simulink model "TDPA"  (R2013a)
settings: Solver=ode3  StartTime=0.0  StopTime=inf  FixedStep=1e-3  RelTol=1e-3
undefined symbols (not defined in the file or in its folder): bDevice, bWall, DBPf, DBPv, kc, Kd, Kp, kWall, mc, mDevice, nWall, POPCM_off, POPCS_off, pos, T1, T2, tSampling, xWall
libraries: quarc_library x2
settings Model: SimulationMode=external  Creator=thaole910  LastModifiedBy=Mech430
settings SolverCC: PositivePriorityOrder=on
settings DebuggingCC: FrameProcessingCompatibilityMsg=error
settings RTWCC: SystemTargetFile=quarc_win64.tlc  TemplateMakefile=quarc_default_tmf  Description=QUARC Win64 Target
settings STFCustomTargetCC: TargetPreCompLibLocation=C:\PROGRA~3\QUARC\lib\2015b\win64\release  CodeReplacementLibrary=C89/C90 (ANSI)  ConcurrentExecutionCompliant=on  GRTInterface=on  SystemTargetFile=quarc_win64.tlc
settings GRTTargetCC: TargetPreCompLibLocation=C:\PROGRA~3\QUARC\lib\2015b\win64\release  CodeReplacementLibrary=C89/C90 (ANSI)  ParMdlRefBuildCompliant=off  CompOptLevelCompliant=off  GeneratePreprocessorConditionals=Use local settings  CombineOutputUpdateFcns=off  MatFileLogging=off  GRTInterface=on  ExtMode=on  ExtModeMexFile=quarc_comm

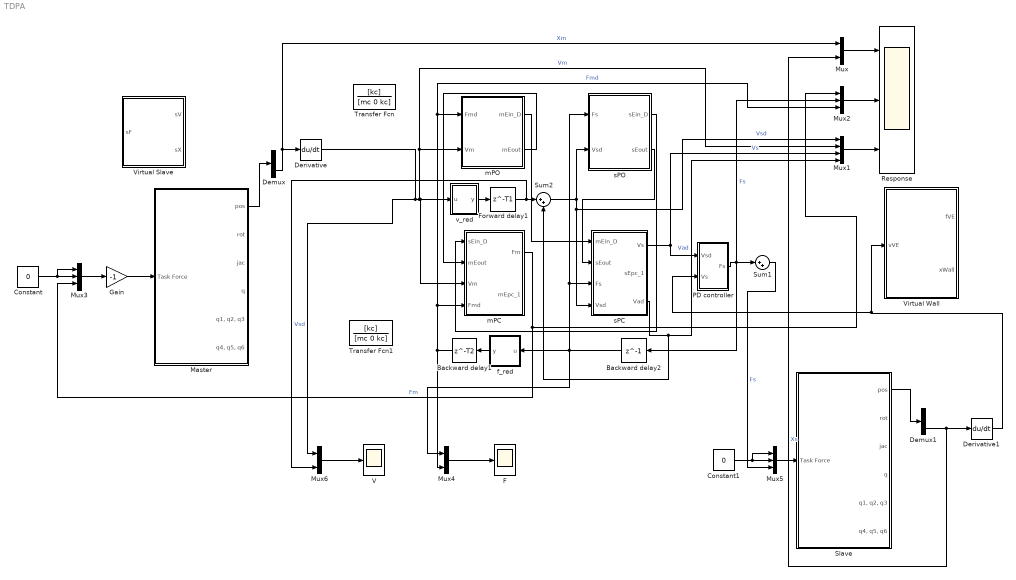
== system TDPA ==
  Backward delay1 : Delay  DelayLength=T2  InitialCondition=0  SampleTime=tSampling
  Backward delay2 : Delay  DelayLength=1  InitialCondition=0  SampleTime=tSampling
  Constant : Constant  Value=0
  Constant1 : Constant  Value=0
  Demux : Demux  Outputs=3
  Demux1 : Demux  Outputs=3
  Derivative : Derivative
  Derivative1 : Derivative
  F : Scope
      settings: TimeRange=100  ShowLegends=on  MaxDataPoints=5000  SaveToWorkspace=off  SaveName=F1  YMin=-4.35585  YMax=15.33258  SampleTime=-1  DataFormat=Array
  Forward delay1 : Delay  DelayLength=T1  InitialCondition=0  SampleTime=tSampling
  Gain : Gain  Gain=-1
  Master : Subsystem
  Mux : Mux  Inputs=2
  Mux1 : Mux
  Mux2 : Mux  Inputs=3
  Mux3 : Mux  Inputs=3
  Mux4 : Mux  Inputs=2
  Mux5 : Mux  Inputs=3
  Mux6 : Mux  Inputs=2
  PD controller : Subsystem
  Response : Scope  NumInputPorts=3
      settings: TimeRange=3.624844027539234  ShowLegends=on  MaxDataPoints=5000  SaveToWorkspace=off  SaveName=ScopeData2  YMin=-0.20269~-3.66024~-1.75917  YMax=0.14159~14.48477~6.94419  SampleInput=on  Decimation=10
  Slave : Subsystem
  Sum1 : Sum  Inputs=|++  SampleTime=tSampling
  Sum2 : Sum  Inputs=|++
  Transfer Fcn : TransferFcn  Numerator=[kc]  Denominator=[mc 0 kc]
  Transfer Fcn1 : TransferFcn  Numerator=[kc]  Denominator=[mc 0 kc]
  V : Scope
      settings: TimeRange=100  ShowLegends=on  MaxDataPoints=5000  SaveToWorkspace=off  SaveName=F  YMin=-1.10119  YMax=1.02242  SampleTime=-1  DataFormat=Array
  Virtual Slave : Subsystem
  Virtual Wall : Subsystem
  f_red : Subsystem
  mPC : Subsystem
  mPO : Subsystem
  sPC : Subsystem
  sPO : Subsystem
  v_red : Subsystem
  wires:
  PD controller/1(Fs) -> Sum1/1, Backward delay2/1, Mux2/2  "Fs"
  Derivative1/1 -> Virtual Wall/1(vVE), PD controller/2(Vs)
  mPO/2(mEout) -> mPC/2(mEout)
  mPO/1(mEin_D) -> sPC/1(mEin_D)
  sPO/1(sEin_D) -> mPC/1(sEin_D)
  sPO/2(sEout) -> sPC/2(sEout)
  Backward delay1/1 -> Mux4/2, mPC/4(Fmd), Mux2/3, mPO/1(Fmd)  "Fmd"
  Backward delay2/1 -> Mux4/1, sPO/1(Fs), sPC/3(Fs), f_red/1(u)
  Mux/1 -> Response/1
  Mux2/1 -> Response/2
  Mux1/1 -> Response/3
  Derivative/1 -> Mux6/1, Mux1/2, mPO/2(Vm), mPC/3(Vm), v_red/1(u)  "Vm"
  mPC/1(Fm) -> Mux3/3, Mux2/1  "Fm"
  Mux4/1 -> F/1
  Forward delay1/1 -> Mux6/2, Sum2/1  "Vsd"
  sPC/3(Vad) -> Sum2/2, Mux1/4  "Vad"
  Sum2/1 -> Mux1/1, sPC/4(Vsd), sPO/2(Vsd)  "Vsd"
  sPC/1(Vs) -> PD controller/1(Vsd), Mux1/3  "Vs"
  Gain/1 -> Master/1(Task Force)
  Master/1(pos) -> Demux/1
  Mux3/1 -> Gain/1
  Constant/1 -> Mux3/2, Mux3/1
  Demux1/3 -> Mux/2, Derivative1/1  "Xs"
  Slave/1(pos) -> Demux1/1
  Mux5/1 -> Slave/1(Task Force)
  Constant1/1 -> Mux5/2, Mux5/1
  Demux/3 -> Mux/1, Derivative/1  "Xm"
  Sum1/1 -> Mux5/3  "Fs"
  v_red/1(y) -> Forward delay1/1
  f_red/1(y) -> Backward delay1/1
  Mux6/1 -> V/1

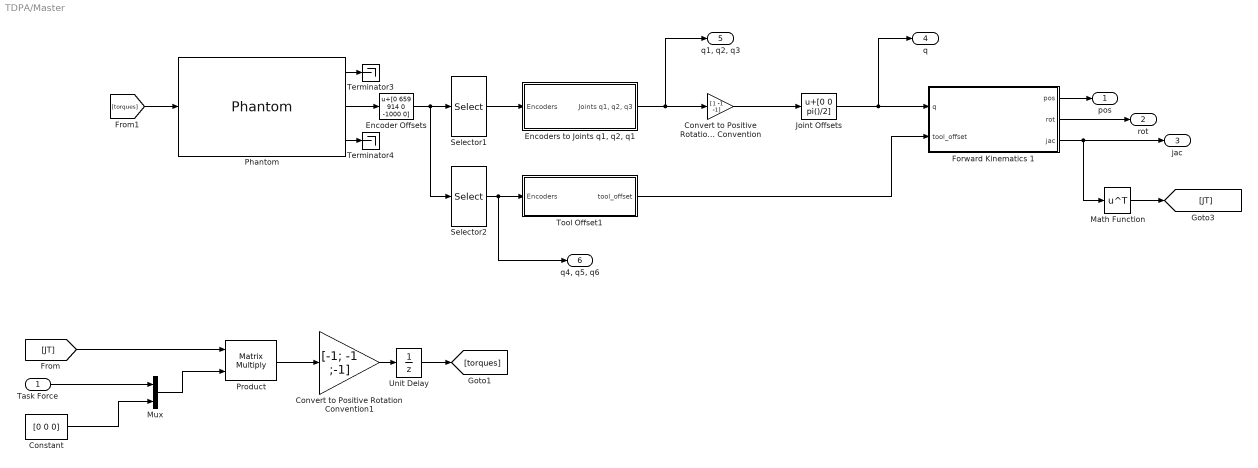
== system TDPA/Master ==
  Task Force : Inport
  Constant : Constant  Value=[0 0 0]
  Convert to Positive Rotation Convention : Gain  Gain=[1 -1 -1]
  Convert to Positive Rotation Convention1 : Gain  Gain=[-1; -1 ;-1]
  Encoder Offsets : Bias  Bias=[0 659 914 0 -1000 0]
  "Encoders to Joints q1, q2, q1" : Subsystem
  Forward Kinematics 1 : MATLAB Function  TreatAsAtomicUnit=on
      settings: PermitHierarchicalResolution=ParametersOnly
  Joint Offsets : Bias  Bias=[0 0 pi()/2]
  Math Function : Math  Operator=transpose  SaturateOnIntegerOverflow=on
  Mux : Mux  Inputs=2
  Phantom : quarc_library/Devices/Third-Party/SensAble/Phantom/Phantom  device_name=Master  output_type=Encoders Values  input_type=Joint space  velocity_limit_option=on  velocity_limit=1200  is_7dof=off  sample_time=-1
      settings: AttributesFormatString=(%<device_name>)
  Product : Product  Multiplication=Matrix(*)  RndMeth=Zero
  Selector1 : Selector  InputPortWidth=6  IndexOptions=Index vector (dialog)  Indices=[1:3]  OutputSizes=1
  Selector2 : Selector  InputPortWidth=6  IndexOptions=Index vector (dialog)  Indices=[4:6]  OutputSizes=1
  Terminator3 : Terminator
  Terminator4 : Terminator
  Tool Offset1 : MATLAB Function  TreatAsAtomicUnit=on
      settings: PermitHierarchicalResolution=ParametersOnly
  Unit Delay : UnitDelay  SampleTime=-1
  pos : Outport
  rot : Outport  Port=2
  jac : Outport  Port=3
  q : Outport  Port=4
  "q1, q2, q3" : Outport  Port=5
  "q4, q5, q6" : Outport  Port=6
  wires:
  Math Function/1 -> [JT]
  Forward Kinematics 1/3(jac) -> Math Function/1, jac/1
  [JT] -> Product/1
  Forward Kinematics 1/1(pos) -> pos/1
  Forward Kinematics 1/2(rot) -> rot/1
  Constant/1 -> Mux/2
  Task Force/1 -> Mux/1
  Mux/1 -> Product/2
  Convert to Positive Rotation Convention/1 -> Joint Offsets/1
  Convert to Positive Rotation Convention1/1 -> Unit Delay/1
  Joint Offsets/1 -> q/1, Forward Kinematics 1/1(q)
  Product/1 -> Convert to Positive Rotation Convention1/1
  Phantom/2 -> Encoder Offsets/1
  [torques] -> Phantom/1
  Phantom/3 -> Terminator4/1
  Phantom/1 -> Terminator3/1
  Selector2/1 -> Tool Offset1/1(Encoders), "q4, q5, q6"/1
  Selector1/1 -> "Encoders to Joints q1, q2, q1"/1(Encoders)
  Encoder Offsets/1 -> Selector1/1, Selector2/1
  "Encoders to Joints q1, q2, q1"/1("Joints q1, q2, q3") -> Convert to Positive Rotation Convention/1, "q1, q2, q3"/1
  Tool Offset1/1(tool_offset) -> Forward Kinematics 1/2(tool_offset)
  Unit Delay/1 -> [torques]

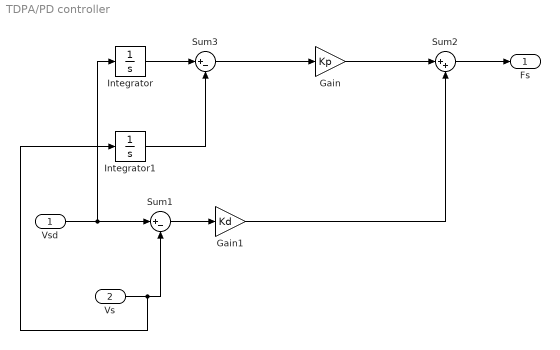
== system TDPA/PD controller ==
  Vsd : Inport
  Vs : Inport  Port=2
  Gain : Gain  Gain=Kp
  Gain1 : Gain  Gain=Kd
  Integrator : Integrator
  Integrator1 : Integrator
  Sum1 : Sum  Inputs=|+-
  Sum2 : Sum  Inputs=|++
  Sum3 : Sum  Inputs=|+-
  Fs : Outport
  wires:
  Sum1/1 -> Gain1/1
  Gain/1 -> Sum2/1
  Vs/1 -> Integrator1/1, Sum1/2
  Gain1/1 -> Sum2/2
  Sum2/1 -> Fs/1
  Sum3/1 -> Gain/1
  Vsd/1 -> Integrator/1, Sum1/1
  Integrator/1 -> Sum3/1
  Integrator1/1 -> Sum3/2

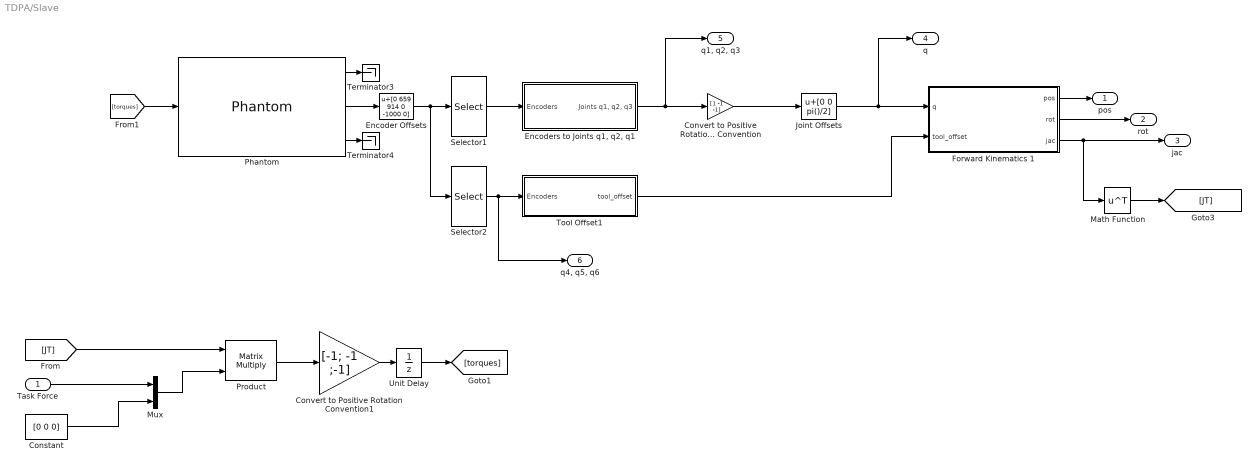
== system TDPA/Slave ==
  Task Force : Inport
  Constant : Constant  Value=[0 0 0]
  Convert to Positive Rotation Convention : Gain  Gain=[1 -1 -1]
  Convert to Positive Rotation Convention1 : Gain  Gain=[-1; -1 ;-1]
  Encoder Offsets : Bias  Bias=[0 659 914 0 -1000 0]
  "Encoders to Joints q1, q2, q1" : Subsystem
  Forward Kinematics 1 : MATLAB Function  TreatAsAtomicUnit=on
      settings: PermitHierarchicalResolution=ParametersOnly
  Joint Offsets : Bias  Bias=[0 0 pi()/2]
  Math Function : Math  Operator=transpose  SaturateOnIntegerOverflow=on
  Mux : Mux  Inputs=2
  Phantom : quarc_library/Devices/Third-Party/SensAble/Phantom/Phantom  device_name=Slave  output_type=Encoders Values  input_type=Joint space  velocity_limit_option=on  velocity_limit=1200  is_7dof=off  sample_time=-1
      settings: AttributesFormatString=(%<device_name>)
  Product : Product  Multiplication=Matrix(*)  RndMeth=Zero
  Selector1 : Selector  InputPortWidth=6  IndexOptions=Index vector (dialog)  Indices=[1:3]  OutputSizes=1
  Selector2 : Selector  InputPortWidth=6  IndexOptions=Index vector (dialog)  Indices=[4:6]  OutputSizes=1
  Terminator3 : Terminator
  Terminator4 : Terminator
  Tool Offset1 : MATLAB Function  TreatAsAtomicUnit=on
      settings: PermitHierarchicalResolution=ParametersOnly
  Unit Delay : UnitDelay  SampleTime=-1
  pos : Outport
  rot : Outport  Port=2
  jac : Outport  Port=3
  q : Outport  Port=4
  "q1, q2, q3" : Outport  Port=5
  "q4, q5, q6" : Outport  Port=6
  wires:
  Math Function/1 -> [JT]
  Forward Kinematics 1/3(jac) -> Math Function/1, jac/1
  [JT] -> Product/1
  Forward Kinematics 1/1(pos) -> pos/1
  Forward Kinematics 1/2(rot) -> rot/1
  Constant/1 -> Mux/2
  Task Force/1 -> Mux/1
  Mux/1 -> Product/2
  Convert to Positive Rotation Convention/1 -> Joint Offsets/1
  Convert to Positive Rotation Convention1/1 -> Unit Delay/1
  Joint Offsets/1 -> q/1, Forward Kinematics 1/1(q)
  Product/1 -> Convert to Positive Rotation Convention1/1
  Phantom/2 -> Encoder Offsets/1
  [torques] -> Phantom/1
  Phantom/3 -> Terminator4/1
  Phantom/1 -> Terminator3/1
  Selector2/1 -> Tool Offset1/1(Encoders), "q4, q5, q6"/1
  Selector1/1 -> "Encoders to Joints q1, q2, q1"/1(Encoders)
  Encoder Offsets/1 -> Selector1/1, Selector2/1
  "Encoders to Joints q1, q2, q1"/1("Joints q1, q2, q3") -> Convert to Positive Rotation Convention/1, "q1, q2, q3"/1
  Tool Offset1/1(tool_offset) -> Forward Kinematics 1/2(tool_offset)
  Unit Delay/1 -> [torques]

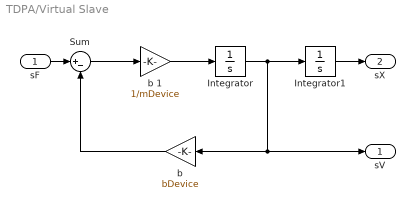
== system TDPA/Virtual Slave ==
  sF : Inport
  Integrator : Integrator  UpperSaturationLimit=10  LowerSaturationLimit=-10
  Integrator1 : Integrator  UpperSaturationLimit=10  LowerSaturationLimit=-10
  Sum : Sum  Inputs=|+-
  "b " : Gain  Gain=bDevice
  b 1 : Gain  Gain=1/mDevice
  sV : Outport
  sX : Outport  Port=2
  wires:
  b 1/1 -> Integrator/1
  sF/1 -> Sum/1
  "b "/1 -> Sum/2
  Sum/1 -> b 1/1
  Integrator/1 -> Integrator1/1, "b "/1, sV/1
  Integrator1/1 -> sX/1

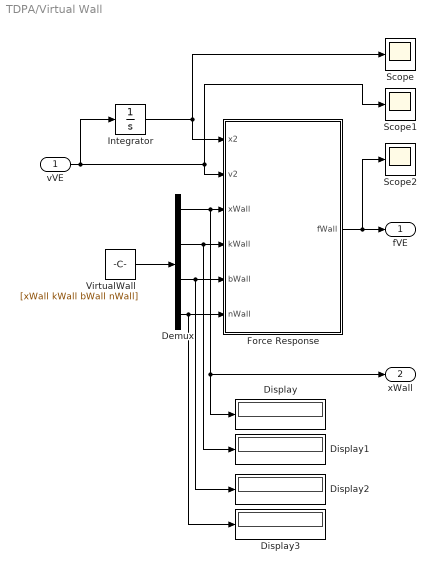
== system TDPA/Virtual Wall ==
  vVE : Inport
  Demux : Demux
  Display{,1..3} (4 alike) : Display
  Force Response : MATLAB Function  TreatAsAtomicUnit=on
      settings: PermitHierarchicalResolution=ParametersOnly
  Integrator : Integrator
  Scope : Scope
      settings: TimeRange=auto  MaxDataPoints=5000  SaveToWorkspace=off  SaveName=ScopeData8  YMin=-10  YMax=10  SampleTime=-1
  Scope1 : Scope
      settings: TimeRange=auto  MaxDataPoints=5000  SaveToWorkspace=off  SaveName=ScopeData9  YMin=-10  YMax=10  SampleTime=-1
  Scope2 : Scope
      settings: TimeRange=auto  MaxDataPoints=5000  SaveToWorkspace=off  SaveName=ScopeData11  YMin=-10  YMax=10  SampleTime=-1
  VirtualWall : Constant  Value=[xWall kWall bWall nWall]  VectorParams1D=off
  fVE : Outport
  xWall : Outport  Port=2
  wires:
  Integrator/1 -> Scope/1, Force Response/1(x2)
  Force Response/1(fWall) -> Scope2/1, fVE/1
  vVE/1 -> Integrator/1, Scope1/1, Force Response/2(v2)
  Demux/1 -> xWall/1, Display/1, Force Response/3(xWall)
  Demux/2 -> Force Response/4(kWall), Display1/1
  Demux/3 -> Display2/1, Force Response/5(bWall)
  Demux/4 -> Force Response/6(nWall), Display3/1
  VirtualWall/1 -> Demux/1

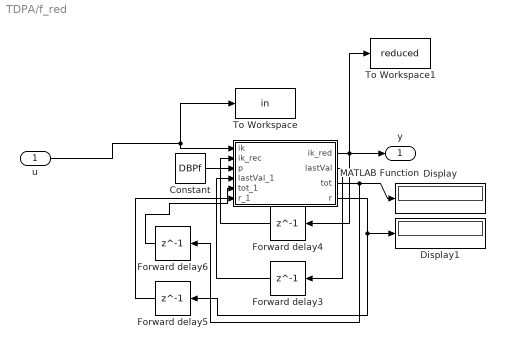
== system TDPA/f_red ==
  u : Inport
  Constant : Constant  Value=DBPf
  Display : Display
  Display1 : Display
  Forward delay{3..6} (4 alike) : Delay  DelayLength=1  InitialCondition=0  InputProcessing=Inherited  SampleTime=tSampling
  MATLAB Function : MATLAB Function  TreatAsAtomicUnit=on
      settings: PermitHierarchicalResolution=ParametersOnly
  To Workspace : ToWorkspace  VariableName=in  SaveFormat=Timeseries  SampleTime=-1
  To Workspace1 : ToWorkspace  VariableName=reduced  SaveFormat=Timeseries  SampleTime=-1
  y : Outport
  wires:
  Forward delay3/1 -> MATLAB Function/4(lastVal_1)
  MATLAB Function/1(ik_red) -> y/1, Forward delay4/1, To Workspace1/1
  Forward delay4/1 -> MATLAB Function/2(ik_rec)
  Constant/1 -> MATLAB Function/3(p)
  MATLAB Function/2(lastVal) -> Forward delay3/1
  MATLAB Function/3(tot) -> Forward delay6/1, Display/1
  Forward delay6/1 -> MATLAB Function/5(tot_1)
  MATLAB Function/4(r) -> Forward delay5/1, Display1/1
  Forward delay5/1 -> MATLAB Function/6(r_1)
  u/1 -> MATLAB Function/1(ik), To Workspace/1

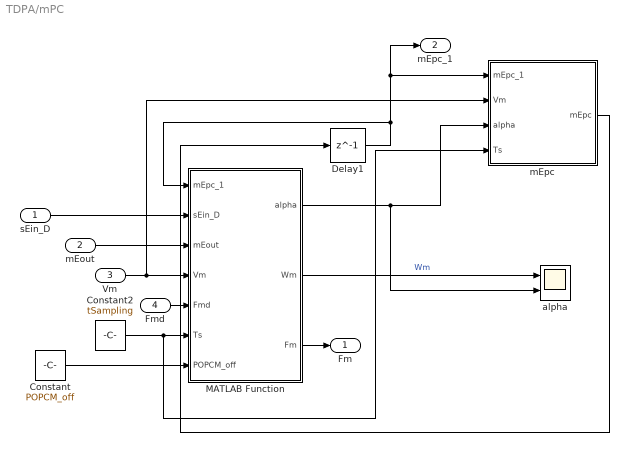
== system TDPA/mPC ==
  sEin_D : Inport
  mEout : Inport  Port=2
  Vm : Inport  Port=3
  Fmd : Inport  Port=4
  Constant : Constant  Value=POPCM_off
  Constant2 : Constant  Value=tSampling
  Delay1 : Delay  DelayLength=1  InitialCondition=0
  MATLAB Function : MATLAB Function  TreatAsAtomicUnit=on
      settings: PermitHierarchicalResolution=ParametersOnly
  alpha : Scope  NumInputPorts=2
      settings: TimeRange=10  ShowLegends=on  MaxDataPoints=5000  SaveToWorkspace=off  SaveName=ScopeData3  YMin=-1~0  YMax=8~3.5  SampleTime=-1
  mEpc : MATLAB Function  TreatAsAtomicUnit=on
      settings: PermitHierarchicalResolution=ParametersOnly
  Fm : Outport
  mEpc_1 : Outport  Port=2
  wires:
  MATLAB Function/1(alpha) -> mEpc/3(alpha), alpha/2
  sEin_D/1 -> MATLAB Function/2(sEin_D)
  Vm/1 -> MATLAB Function/4(Vm), mEpc/2(Vm)
  mEpc/1(mEpc) -> Delay1/1
  mEout/1 -> MATLAB Function/3(mEout)
  MATLAB Function/3(Fm) -> Fm/1
  Fmd/1 -> MATLAB Function/5(Fmd)
  Constant2/1 -> mEpc/4(Ts), MATLAB Function/6(Ts)
  Delay1/1 -> mEpc/1(mEpc_1), mEpc_1/1, MATLAB Function/1(mEpc_1)
  MATLAB Function/2(Wm) -> alpha/1  "Wm"
  Constant/1 -> MATLAB Function/7(POPCM_off)

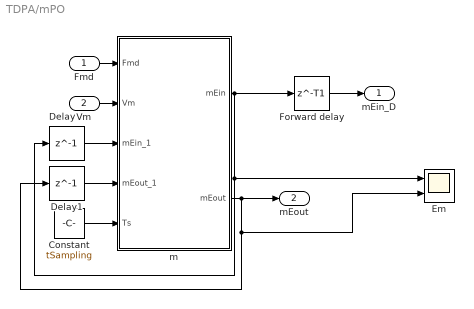
== system TDPA/mPO ==
  Fmd : Inport
  Vm : Inport  Port=2
  Constant : Constant  Value=tSampling
  Delay : Delay  DelayLength=1  InitialCondition=0  SampleTime=tSampling
  Delay1 : Delay  DelayLength=1  InitialCondition=0  SampleTime=tSampling
  Em : Scope  NumInputPorts=2
      settings: TimeRange=auto  ShowLegends=on  MaxDataPoints=5000  SaveToWorkspace=off  SaveName=ScopeData  YMin=-5~-5  YMax=5~5  SampleTime=-1
  Forward delay : Delay  DelayLength=T1  InitialCondition=0  SampleTime=tSampling
  m : MATLAB Function  TreatAsAtomicUnit=on
      settings: PermitHierarchicalResolution=ParametersOnly
  mEin_D : Outport
  mEout : Outport  Port=2
  wires:
  Delay1/1 -> m/4(mEout_1)
  Constant/1 -> m/5(Ts)
  m/2(mEout) -> Em/2, Delay1/1, mEout/1
  Fmd/1 -> m/1(Fmd)
  Vm/1 -> m/2(Vm)
  Delay/1 -> m/3(mEin_1)
  m/1(mEin) -> Em/1, Delay/1, Forward delay/1
  Forward delay/1 -> mEin_D/1

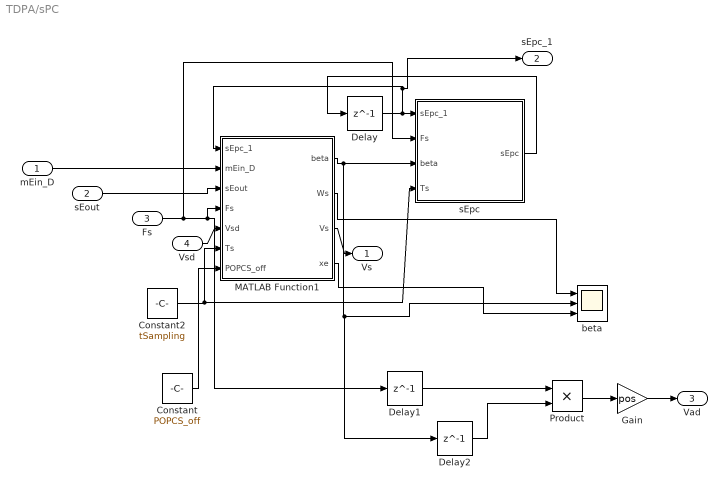
== system TDPA/sPC ==
  mEin_D : Inport
  sEout : Inport  Port=2
  Fs : Inport  Port=3
  Vsd : Inport  Port=4
  Constant : Constant  Value=POPCS_off
  Constant2 : Constant  Value=tSampling
  Delay : Delay  DelayLength=1  InitialCondition=0
  Delay1 : Delay  DelayLength=1  InitialCondition=0
  Delay2 : Delay  DelayLength=1  InitialCondition=0
  Gain : Gain  Gain=pos
  MATLAB Function1 : MATLAB Function  TreatAsAtomicUnit=on
      settings: PermitHierarchicalResolution=ParametersOnly
  Product : Product
  beta : Scope  NumInputPorts=3
      settings: TimeRange=8.70967741935484  ShowLegends=on  MaxDataPoints=5000  SaveToWorkspace=off  SaveName=ScopeData4  YMin=-8~0~-0.5736994219653178  YMax=2~14000~0.02514450867052043  SampleTime=-1
  sEpc : MATLAB Function  TreatAsAtomicUnit=on
      settings: PermitHierarchicalResolution=ParametersOnly
  Vs : Outport
  sEpc_1 : Outport  Port=2
  Vad : Outport  Port=3
  wires:
  Delay/1 -> sEpc_1/1, MATLAB Function1/1(sEpc_1), sEpc/1(sEpc_1)
  MATLAB Function1/3(Vs) -> Vs/1
  Fs/1 -> sEpc/2(Fs), Delay1/1, MATLAB Function1/4(Fs)
  mEin_D/1 -> MATLAB Function1/2(mEin_D)
  Constant2/1 -> MATLAB Function1/6(Ts), sEpc/4(Ts)
  Vsd/1 -> MATLAB Function1/5(Vsd)
  sEout/1 -> MATLAB Function1/3(sEout)
  MATLAB Function1/1(beta) -> Delay2/1, beta/2, sEpc/3(beta)
  MATLAB Function1/2(Ws) -> beta/1
  sEpc/1(sEpc) -> Delay/1
  Constant/1 -> MATLAB Function1/7(POPCS_off)
  Product/1 -> Gain/1
  Delay1/1 -> Product/1
  Delay2/1 -> Product/2
  Gain/1 -> Vad/1
  MATLAB Function1/4(xe) -> beta/3

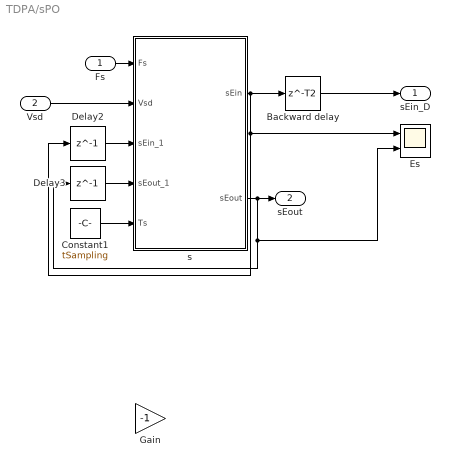
== system TDPA/sPO ==
  Fs : Inport
  Vsd : Inport  Port=2
  Backward delay : Delay  DelayLength=T2  InitialCondition=0  SampleTime=tSampling
  Constant1 : Constant  Value=tSampling
  Delay2 : Delay  DelayLength=1  InitialCondition=0  SampleTime=tSampling
  Delay3 : Delay  DelayLength=1  InitialCondition=0  SampleTime=tSampling
  Es : Scope  NumInputPorts=2
      settings: TimeRange=auto  ShowLegends=on  MaxDataPoints=5000  SaveToWorkspace=off  YMin=-5~-5  YMax=5~5  SampleTime=-1
  Gain : Gain  Gain=-1
  s : MATLAB Function  TreatAsAtomicUnit=on
      settings: PermitHierarchicalResolution=ParametersOnly
  sEin_D : Outport
  sEout : Outport  Port=2
  wires:
  Fs/1 -> s/1(Fs)
  s/2(sEout) -> Es/2, Delay3/1, sEout/1
  Delay2/1 -> s/3(sEin_1)
  Constant1/1 -> s/5(Ts)
  Delay3/1 -> s/4(sEout_1)
  s/1(sEin) -> Es/1, Delay2/1, Backward delay/1
  Vsd/1 -> s/2(Vsd)
  Backward delay/1 -> sEin_D/1

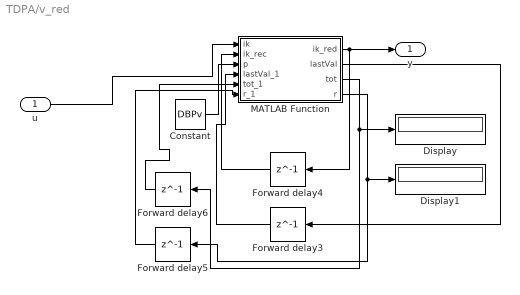
== system TDPA/v_red ==
  u : Inport
  Constant : Constant  Value=DBPv
  Display : Display
  Display1 : Display
  Forward delay{3..6} (4 alike) : Delay  DelayLength=1  InitialCondition=0  InputProcessing=Inherited  SampleTime=tSampling
  MATLAB Function : MATLAB Function  TreatAsAtomicUnit=on
      settings: PermitHierarchicalResolution=ParametersOnly
  y : Outport
  wires:
  Forward delay3/1 -> MATLAB Function/4(lastVal_1)
  MATLAB Function/1(ik_red) -> y/1, Forward delay4/1
  Forward delay4/1 -> MATLAB Function/2(ik_rec)
  Constant/1 -> MATLAB Function/3(p)
  u/1 -> MATLAB Function/1(ik)
  MATLAB Function/2(lastVal) -> Forward delay3/1
  MATLAB Function/3(tot) -> Forward delay6/1, Display/1
  Forward delay6/1 -> MATLAB Function/5(tot_1)
  MATLAB Function/4(r) -> Forward delay5/1, Display1/1
  Forward delay5/1 -> MATLAB Function/6(r_1)

== system TDPA/Master/Encoders to Joints q1, q2, q1 ==
  Encoders : Inport
  Bias1 : Bias  Bias=[0 -659 -910]
  Embedded MATLAB Function : MATLAB Function  TreatAsAtomicUnit=on
      settings: PermitHierarchicalResolution=ParametersOnly
  Encoder : Gain  Gain=2*pi/2048
  Gear Ratio : Gain  Gain=1./[7.461 -7.519 7.529]
  "Joints q1, q2, q3" : Outport
  wires:
  Embedded MATLAB Function/1(q) -> "Joints q1, q2, q3"/1
  Encoders/1 -> Bias1/1
  Encoder/1 -> Gear Ratio/1
  Gear Ratio/1 -> Embedded MATLAB Function/1(m)
  Bias1/1 -> Encoder/1

== system TDPA/Slave/Encoders to Joints q1, q2, q1 ==
  Encoders : Inport
  Bias1 : Bias  Bias=[0 -659 -910]
  Embedded MATLAB Function : MATLAB Function  TreatAsAtomicUnit=on
      settings: PermitHierarchicalResolution=ParametersOnly
  Encoder : Gain  Gain=2*pi/2048
  Gear Ratio : Gain  Gain=1./[7.461 -7.519 7.529]
  "Joints q1, q2, q3" : Outport
  wires:
  Embedded MATLAB Function/1(q) -> "Joints q1, q2, q3"/1
  Encoders/1 -> Bias1/1
  Encoder/1 -> Gear Ratio/1
  Gear Ratio/1 -> Embedded MATLAB Function/1(m)
  Bias1/1 -> Encoder/1

== matlab function TDPA/sPO/s ==
  data: Fs input; sEin output; Vsd input; sEin_1 input; sEout_1 input; Ts input; sEout output
function[sEin,sEout] = fcn(Fs,Vsd,sEin_1,sEout_1,Ts)
dE = Fs*Vsd*Ts;
    if dE > 0
        sEin = sEin_1;
        sEout = sEout_1 + dE;
    else
        sEin = sEin_1 - dE;
        sEout = sEout_1;
    end
end

== matlab function TDPA/mPO/m ==
  data: Fmd input; mEin output; Vm input; mEin_1 input; mEout_1 input; Ts input; mEout output
function[mEin,mEout] = fcn(Fmd,Vm,mEin_1,mEout_1,Ts)
dE = Fmd*Vm*Ts;
    if dE > 0
        mEin = mEin_1 + dE;
        mEout = mEout_1;
    else
        mEin = mEin_1;
        mEout = mEout_1 - dE;
    end
end

== matlab function TDPA/Slave/Encoders to Joints q1, q2, q1/Embedded MATLAB Function ==
  data: m input; q output
function q = Motors_2_Joints(m)
q = m;
q(1) = m(1);
q(2) = m(2);
q(3) = m(3) - m(2) -pi/2;
end

== matlab function TDPA/sPC/sEpc ==
  data: sEpc_1 input; sEpc output; Fs input; beta input; Ts input
function sEpc = fcn(sEpc_1,Fs,beta,Ts)
    sEpc = Fs^2*beta*Ts +  sEpc_1;
end

== matlab function TDPA/mPC/mEpc ==
  data: mEpc_1 input; Vm input; alpha input; Ts input; mEpc output
function mEpc = fcn(mEpc_1,Vm,alpha,Ts)
    mEpc =  Vm^2*alpha*Ts + mEpc_1;
end

== matlab function TDPA/mPC/MATLAB Function ==
  data: mEpc_1 input; sEin_D input; alpha output; mEout input; Wm output; Vm input; Fmd input; Ts input; Fm output; POPCM_off input
function [alpha,Wm,Fm] = fcn(mEpc_1,sEin_D,mEout,Vm,Fmd,Ts,POPCM_off)
    Wm = sEin_D - mEout + mEpc_1;
    if (Wm < 0) && (abs(Vm) > 0)
        alpha = - Wm/(Ts*Vm^2);
    else
        alpha = 0;
    end
    if (POPCM_off)
        alpha = 0;
    end
    Fm = Fmd + alpha*Vm;
end

== matlab function TDPA/sPC/MATLAB Function1 ==
  data: sEpc_1 input; mEin_D input; beta output; sEout input; Ws output; Fs input; Vsd input; Ts input; Vs output; POPCS_off input; xe output
function [beta,Ws,Vs,xe] = fcn(sEpc_1,mEin_D,sEout,Fs,Vsd,Ts,POPCS_off)
    Ws = mEin_D - sEout + sEpc_1;
    if (Ws < 0) && (abs(Fs) > 0)
        beta = -Ws/(Ts*Fs^2);
    else
        beta = 0;
    end
    if (POPCS_off)
        beta = 0;
    end
    Vs = Vsd - beta*Fs;
    xe =  -beta*Fs*Ts;
end

== matlab function TDPA/Virtual Wall/Force Response ==
  data: x2 input; fWall output; v2 input; xWall input; kWall input; bWall input; nWall input
function fWall = fcn(x2,v2,xWall,kWall,bWall,nWall)
if ((x2-xWall)'*nWall < 0) 
    fWall = -kWall*((x2-xWall)'*nWall)*nWall - bWall*((v2'*nWall)*nWall);
    if fWall'*nWall < 0 
        fWall = 0;
    end
else
    fWall =0;
end

== matlab function TDPA/Slave/Forward Kinematics 1 ==
  data: pos output; q input; rot output; tool_offset input; jac output
function [pos,rot,jac]    = ForwardKinematics(q,tool_offset)
% This block supports the Embedded MATLAB subset.
% See the help menu for details. 

% Link lengths
L1 = .132;
L2 = .132;

%Define A-matrices
%A1= DH(theta ,d ,a ,alpha)
A1 = DH(q(1), 0, 0, -pi()/2);
A2 = DH(q(2), 0, L1, 0);
A3 = DH(q(3)-pi/2, 0, L2, 0);

%Define T Matrices
T01=A1;
T02=T01*A2;
T03=T02*A3;

%tool_offset given with respect to frame 3.
T_tool=T03*tool_offset;
rot=T_tool(1:3,1:3);
pos=T_tool(1:3,4);

%Axes of rotation in base coordinates. 
z0=[0 0 1]';
z1=T01(1:3,3);
z2=T02(1:3,3);

%Coordinate Frame origins in Base frame coordinates
p0=[0 0 0]';
p1=T01(1:3,4);
p2=T02(1:3,4);
p3=T03(1:3,4);

%Formulation of the Jacobian

%%%%%%%%%%%%%%%%%%%%%%%%%%%%JACOBIAN%%%%%%%%%%%%%%%%%%%%%%%%
jac = [cross(z0,(pos-p0)) cross(z1,(pos-p1)) cross(z2,(pos-p2))
    z0 z1 z2];

end

function A = DH(theta, d, a, alpha)

A_R_z = [cos(theta) -sin(theta) 0 0;
         sin(theta) cos(theta) 0 0;
         0 0 1 0;
         0 0 0 1];

A_T_z = [1 0 0 0;
         0 1 0 0;
         0 0 1 d;
         0 0 0 1];
     
  

A_T_x = [1 0 0 a;
         0 1 0 0;
         0 0 1 0;
         0 0 0 1];

A_R_x = [1 0 0 0;
         0 cos(alpha) -sin(alpha)  0;
         0 sin(alpha) cos(alpha) 0;
         0 0 0 1];

A = A_R_z*A_T_z*A_T_x*A_R_x;

end

== matlab function TDPA/Master/Encoders to Joints q1, q2, q1/Embedded MATLAB Function ==
  data: m input; q output
function q = Motors_2_Joints(m)
q = m;
q(1) = m(1);
q(2) = m(2);
q(3) = m(3) - m(2) -pi/2;
end

== matlab function TDPA/Master/Forward Kinematics 1 ==
  data: pos output; q input; rot output; tool_offset input; jac output
function [pos,rot,jac]    = ForwardKinematics(q,tool_offset)
% This block supports the Embedded MATLAB subset.
% See the help menu for details. 

% Link lengths
L1 = .132;
L2 = .132;

%Define A-matrices
%A1= DH(theta ,d ,a ,alpha)
A1 = DH(q(1), 0, 0, -pi()/2);
A2 = DH(q(2), 0, L1, 0);
A3 = DH(q(3)-pi/2, 0, L2, 0);

%Define T Matrices
T01=A1;
T02=T01*A2;
T03=T02*A3;

%tool_offset given with respect to frame 3.
T_tool=T03*tool_offset;
rot=T_tool(1:3,1:3);
pos=T_tool(1:3,4);

%Axes of rotation in base coordinates. 
z0=[0 0 1]';
z1=T01(1:3,3);
z2=T02(1:3,3);

%Coordinate Frame origins in Base frame coordinates
p0=[0 0 0]';
p1=T01(1:3,4);
p2=T02(1:3,4);
p3=T03(1:3,4);

%Formulation of the Jacobian

%%%%%%%%%%%%%%%%%%%%%%%%%%%%JACOBIAN%%%%%%%%%%%%%%%%%%%%%%%%
jac = [cross(z0,(pos-p0)) cross(z1,(pos-p1)) cross(z2,(pos-p2))
    z0 z1 z2];

end

function A = DH(theta, d, a, alpha)

A_R_z = [cos(theta) -sin(theta) 0 0;
         sin(theta) cos(theta) 0 0;
         0 0 1 0;
         0 0 0 1];

A_T_z = [1 0 0 0;
         0 1 0 0;
         0 0 1 d;
         0 0 0 1];
     
  

A_T_x = [1 0 0 a;
         0 1 0 0;
         0 0 1 0;
         0 0 0 1];

A_R_x = [1 0 0 0;
         0 cos(alpha) -sin(alpha)  0;
         0 sin(alpha) cos(alpha) 0;
         0 0 0 1];

A = A_R_z*A_T_z*A_T_x*A_R_x;

end

== matlab function TDPA/Master/Tool Offset1 ==
  data: Encoders input; tool_offset output
function tool_offset = getToolOffset(Encoders)

%convert encoder values to angles using bias and gain
bias = [-2048 -2654 -2048];
gain = [2*pi()/4915 2*pi()/4096 2*pi()/4915];
Angle = (Encoders' + bias).*gain;

% convert the angle to the positive rotation convention defined
% by DH parameters
pos_rot = [-1 1 1];
joint_offset = [0 -(40-180)*pi/180 0];
Joint456 = Angle.*pos_rot + joint_offset;

%pick off theta4 and theta5
theta4 = Joint456(1);
theta5 = Joint456(2);

% The orientation of the tool offset matrix is given two successive
% rotations about x and z axis. 
RotZ = [cos(theta5) -sin(theta5) 0; sin(theta5) cos(theta5) 0; 0 0 1];
RotX = [1 0 0; 0 cos(theta4) -sin(theta4); 0 sin(theta4) cos(theta4)];
R = RotX*RotZ; % R is the rotation matrix of the tool offset matrix with respect to frame 3

% with respect to frame 3, the tool is 0.039m in the x-direction. Convert
% this vector to tool frame coordinates
tool_pos =R * [.039; 0; 0];

%create a Tool_offset transformation matrix. Use Identity matrix for
%rotation to show that the end effector frame and frame 3 are always
%aligned
I = [1 0 0; 0 1 0; 0 0 1];
tool = cat(2,I,tool_pos);
tool_offset = cat(1,tool,[0 0 0 1]);

== matlab function TDPA/Slave/Tool Offset1 ==
  data: Encoders input; tool_offset output
function tool_offset = getToolOffset(Encoders)

%convert encoder values to angles using bias and gain
bias = [-2048 -2654 -2048];
gain = [2*pi()/4915 2*pi()/4096 2*pi()/4915];
Angle = (Encoders' + bias).*gain;

% convert the angle to the positive rotation convention defined
% by DH parameters
pos_rot = [-1 1 1];
joint_offset = [0 -(40-180)*pi/180 0];
Joint456 = Angle.*pos_rot + joint_offset;

%pick off theta4 and theta5
theta4 = Joint456(1);
theta5 = Joint456(2);

% The orientation of the tool offset matrix is given two successive
% rotations about x and z axis. 
RotZ = [cos(theta5) -sin(theta5) 0; sin(theta5) cos(theta5) 0; 0 0 1];
RotX = [1 0 0; 0 cos(theta4) -sin(theta4); 0 sin(theta4) cos(theta4)];
R = RotX*RotZ; % R is the rotation matrix of the tool offset matrix with respect to frame 3

% with respect to frame 3, the tool is 0.039m in the x-direction. Convert
% this vector to tool frame coordinates
tool_pos =R * [.039; 0; 0];

%create a Tool_offset transformation matrix. Use Identity matrix for
%rotation to show that the end effector frame and frame 3 are always
%aligned
I = [1 0 0; 0 1 0; 0 0 1];
tool = cat(2,I,tool_pos);
tool_offset = cat(1,tool,[0 0 0 1]);

== matlab function TDPA/v_red/MATLAB Function ==
  data: ik input; ik_red output; ik_rec input; p input; lastVal_1 input; lastVal output; tot output; r output; tot_1 input; r_1 input
function [ik_red,lastVal,tot,r]= fcn(ik,ik_rec,p,lastVal_1,tot_1,r_1)
DB = p*ik;
lastVal = lastVal_1;
if ik_rec ~= 0
    lastVal = ik_rec;
end
if abs(ik-lastVal) >= DB
    ik_red = ik;
    r = r_1;
else
    ik_red = lastVal;
    r = r_1 + 1;
end
tot = tot_1 + 1;

== matlab function TDPA/f_red/MATLAB Function ==
  data: ik input; ik_red output; ik_rec input; p input; lastVal_1 input; lastVal output; tot output; r output; tot_1 input; r_1 input
function [ik_red,lastVal,tot,r]= fcn(ik,ik_rec,p,lastVal_1,tot_1,r_1)
DB = p*ik;
lastVal = lastVal_1;
if ik_rec ~= 0
    lastVal = ik_rec;
end
if abs(ik-lastVal) >= DB
    ik_red = ik;
    r = r_1;
else
    ik_red = lastVal;
    r = r_1 + 1;
end
tot = tot_1 + 1;
